simulink model "linearny_regulator"  (R2021b)
settings: Solver=VariableStepAuto  StartTime=0.0  StopTime=100  MaxStep=1e-2  RelTol=1e-3
undefined symbols (not defined in the file): am, bm, pGain, pT, theta1_ideal, theta2_ideal, upb, ypb
settings Model: Creator=miso  LastModifiedBy=miso

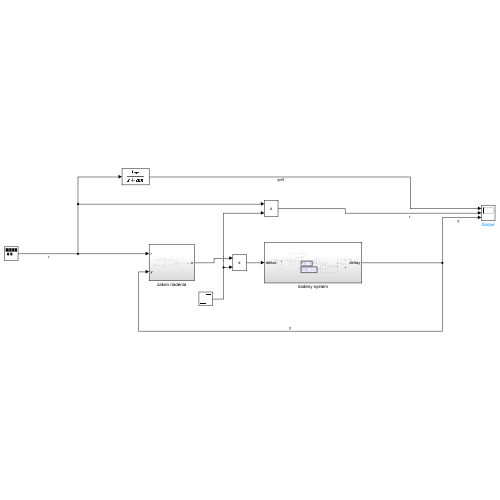
[thumbnail: Simulink's stored preview of the top-level diagram]
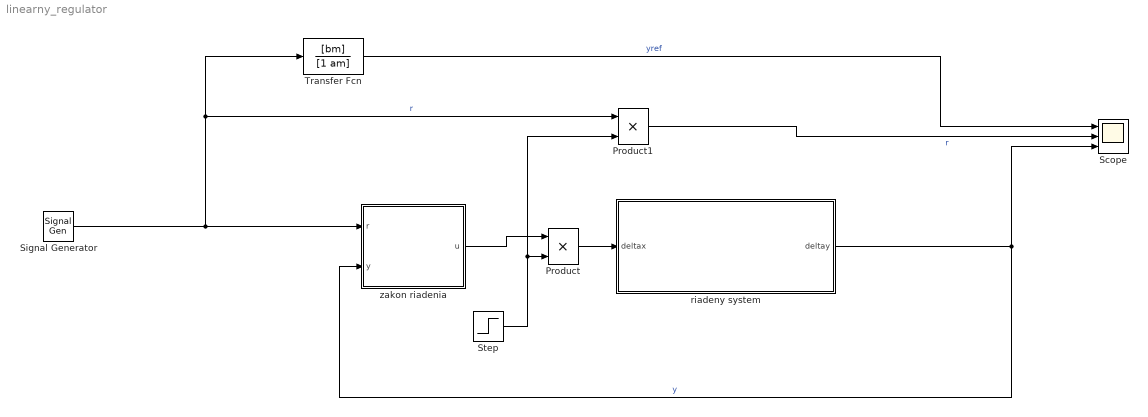
== system linearny_regulator ==
  Product : Product
  Product1 : Product
  Scope : Scope  NumInputPorts=3
  Signal Generator : SignalGenerator  WaveForm=square  Amplitude=-6  Frequency=1/10
  Step : Step  Time=10  SampleTime=0
  Transfer Fcn : TransferFcn  Numerator=[bm]  Denominator=[1 am]
  riadeny system : Subsystem
  zakon riadenia : Subsystem
  wires:
  riadeny system/1(deltay) -> zakon riadenia/2(y), Scope/3  "y"
  Signal Generator/1 -> Transfer Fcn/1, Product1/1, zakon riadenia/1(r)  "r"
  zakon riadenia/1(u) -> Product/1
  Product/1 -> riadeny system/1(deltax)
  Step/1 -> Product1/2, Product/2
  Product1/1 -> Scope/2  "r"
  Transfer Fcn/1 -> Scope/1  "yref"

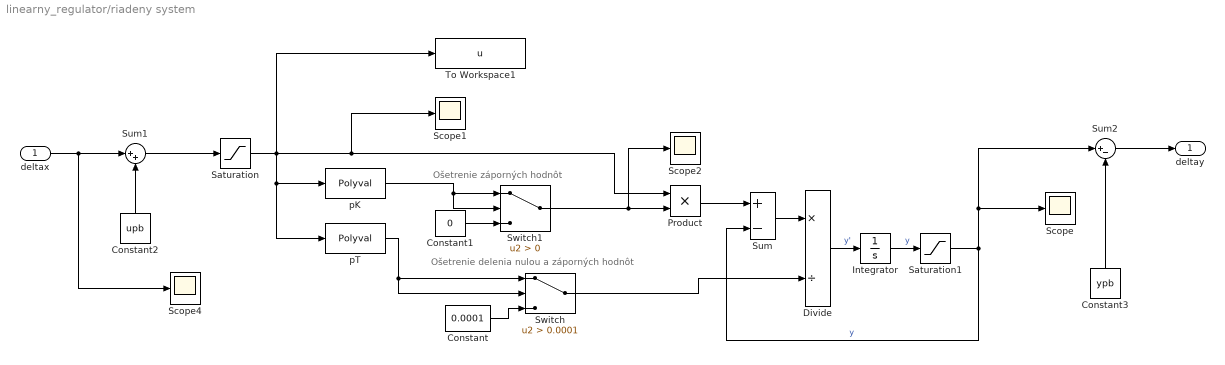
== system linearny_regulator/riadeny system ==
  note: Ošetrenie delenia nulou a záporných hodnôt
  note: Ošetrenie záporných hodnôt
  deltax : Inport
  Constant : Constant  Value=0.0001
  Constant1 : Constant  Value=0
  Constant2 : Constant  Value=upb
  Constant3 : Constant  Value=ypb
  Divide : Product  Inputs=*/
  Integrator : Integrator
  Product : Product
  Saturation : Saturate  UpperLimit=255  LowerLimit=0
  Saturation1 : Saturate  UpperLimit=1023  LowerLimit=0
  Scope{,1..2,4} (4 alike) : Scope
  Sum : Sum  Inputs=+-
  Sum1 : Sum  Inputs=|++
  Sum2 : Sum  Inputs=|+-
  Switch : Switch  Criteria=u2 > Threshold  Threshold=0.0001
  Switch1 : Switch  Criteria=u2 > Threshold
  To Workspace1 : ToWorkspace  VariableName=u  SaveFormat=Timeseries  SampleTime=-1
  pK : Polyval  Coefs=pGain
  pT : Polyval  Coefs=pT
  deltay : Outport
  wires:
  Sum/1 -> Divide/1
  Saturation1/1 -> Sum2/1, Scope/1, Sum/2  "y"
  Constant/1 -> Switch/3
  pT/1 -> Switch/1, Switch/2
  pK/1 -> Switch1/2, Switch1/1
  Switch/1 -> Divide/2
  Constant1/1 -> Switch1/3
  Product/1 -> Sum/1
  Switch1/1 -> Scope2/1, Product/2
  Integrator/1 -> Saturation1/1  "y"
  Divide/1 -> Integrator/1  "y'"
  deltax/1 -> Scope4/1, Sum1/1
  Sum1/1 -> Saturation/1
  Saturation/1 -> To Workspace1/1, pT/1, pK/1, Scope1/1, Product/1
  Constant2/1 -> Sum1/2
  Sum2/1 -> deltay/1
  Constant3/1 -> Sum2/2

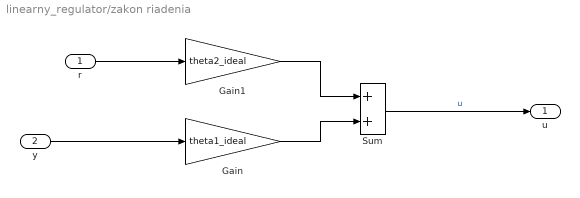
== system linearny_regulator/zakon riadenia ==
  r : Inport
  y : Inport  Port=2
  Gain : Gain  Gain=theta1_ideal
  Gain1 : Gain  Gain=theta2_ideal
  Sum : Sum
  u : Outport
  wires:
  Gain1/1 -> Sum/1
  Gain/1 -> Sum/2
  y/1 -> Gain/1
  Sum/1 -> u/1  "u"
  r/1 -> Gain1/1
